simulink model "buck_boost_model"  (R2022a)
settings: Solver=VariableStepAuto  StartTime=0.0  StopTime=0.007  RelTol=1e-3  AbsTol=1e-3
undefined symbols (not defined in the file or in its folder): dutyCycleTs, init_action
libraries: fl_lib x5, nesl_utility x5, ee_lib x3, checkpacklib x1, dspmathops x1, simulink x1, rllib x1
settings Model: Creator=kevin  LastModifiedBy=kevin
settings SolverCC: AutoScaleAbsTol=off  MaxConsecutiveMinStep=2  AlgebraicLoopSolver=TrustRegion
settings DataIOCC: SaveOutput=off  SignalLogging=off  DSMLogging=off  SaveTime=off  ReturnWorkspaceOutputs=off
settings DebuggingCC: UnconnectedInputMsg=warning  UnconnectedOutputMsg=warning  UnconnectedLineMsg=warning  SymbolicDimsDataTypeCodeGenerationDiagnostic=none  SFMachineParentedDataDiag=warning
settings SFSimCC: CustomCodeUndefinedFunction=UseInterfaceOnly
settings RTWCC: DLArmComputeVersion=19.05
settings SimscapeCC: SimscapeLogSimulationStatistics=on  SimscapeLogDataHistory=10000

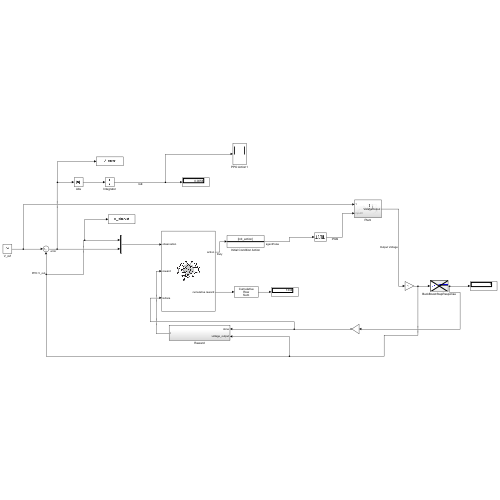
[thumbnail: Simulink's stored preview of the top-level diagram]
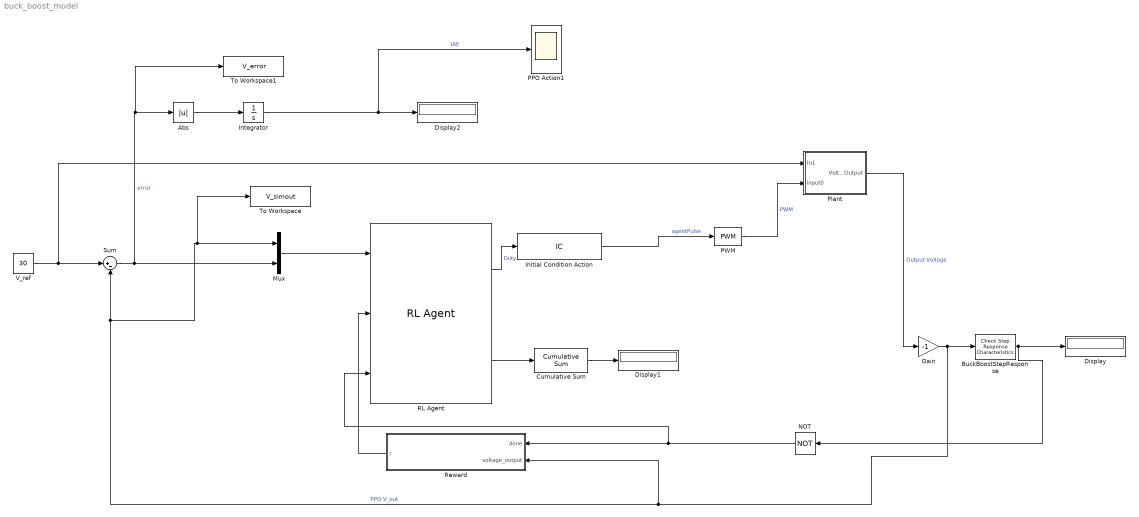
== system buck_boost_model ==
  Abs : Abs  SaturateOnIntegerOverflow=off
  BuckBoostStepResponse : checkpacklib/Check Step Response  Characteristics  InstantiateOnLoad=on  enabled=off  stopWhenAssertionFail=off  export=on  ViewDlgPos=[1.8 41.8 766.4 740.8]  OpenViewOnLoad=off  LaunchViewOnOpen=off  TimeUnits=seconds  EnableStepResponseBound=on  InitialValue=0  FinalValue=30  StepTime=0  RiseTime=0.007  PercentRise=50  SettlingTime=0.0071  PercentSettling=2  PercentOvershoot=30  PercentUndershoot=2
      settings: SourceProductBaseCode=MT,CT,ID,SO
  Cumulative Sum : dspmathops/Cumulative Sum  dim=Rows  InputProcessing=Columns as channels (frame based)  reset_popup=None  roundingMode=Floor  overflowMode=off  outputDataTypeStr=Inherit: Same as accumulator  outputMin=[]  outputMax=[]  outputLastDataTypeStr=Inherit: Same as accumulator
  Display : Display
  Display1 : Display
  Display2 : Display
  Gain : Gain  Gain=-1
  Initial Condition Action : InitialCondition  Value=init_action
  Integrator : Integrator
  Mux : Mux  Inputs=2
  NOT : Logic  Operator=NOT  IconShape=distinctive  AllPortsSameDT=off  OutDataTypeStr=boolean
  PPO Action1 : Scope
  PWM : simulink/Discontinuities/PWM  DisableCoverage=on  Period=1/100000  DisallowZeroDutyCycle=on  RunAtFixedTimeIntervals=off  SampleTime=dutyCycleTs
  Plant : Subsystem
  RL Agent : rllib/RL Agent  Agent=agent  ExternalActionAsInput=off  ProvideLastAction=off  ProvideCumRwd=on  TreatAsDirectFeedthrough=on  UseStrictObservationDataTypes=off
  Reward : Subsystem
  Sum : Sum  Inputs=|+-
  To Workspace : ToWorkspace  VariableName=V_simout  SaveFormat=Timeseries  SampleTime=-1
  To Workspace1 : ToWorkspace  VariableName=V_error  SaveFormat=Timeseries  SampleTime=-1
  V_ref : Constant  Value=30
  wires:
  Plant/1(VoltageOutput) -> Gain/1  "Output Voltage"
  V_ref/1 -> Plant/1(In1), Sum/1
  Mux/1 -> RL Agent/1
  Gain/1 -> To Workspace/1, Mux/1, Sum/2, Reward/2(voltage_output), BuckBoostStepResponse/1  "PPO V_out"
  Sum/1 -> To Workspace1/1, Abs/1, Mux/2  "error"
  Reward/1(r) -> RL Agent/2
  NOT/1 -> Reward/1(done), RL Agent/3
  RL Agent/1 -> Initial Condition Action/1  "Duty"
  RL Agent/2 -> Cumulative Sum/1
  Cumulative Sum/1 -> Display1/1
  Initial Condition Action/1 -> PWM/1  "agentPulse"
  PWM/1 -> Plant/2(input0)  "PWM"
  BuckBoostStepResponse/1 -> NOT/1, Display/1
  Abs/1 -> Integrator/1
  Integrator/1 -> PPO Action1/1, Display2/1  "IAE"

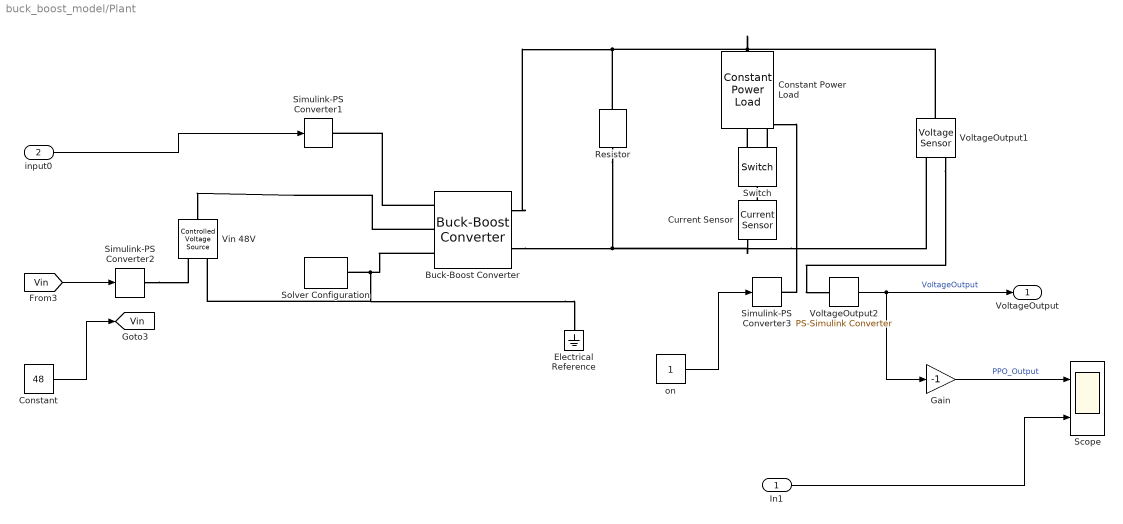
== system buck_boost_model/Plant ==
  In1 : Inport
  input0 : Inport  Port=2
  Buck-Boost Converter : ee_lib/Semiconductors & Converters/Converters/Buck-Boost Converter  device_type=ee.enum.converters.switchingdevice.mosfet  Vf=0.8 V  Ron=0.001 Ohm  Rds=1e-3 Ohm  Goff=1e-3 1/Ohm  Vth=0.0001 V  Vgt=1 V  Vgt_off=-1 V  Ih=1 A  diode_param=ee.enum.converters.diode.nodynamics  diode_Vf=0.00001 V  diode_Ron=1e-3 Ohm  diode_Goff=1e-5 1/Ohm  diode_C=50 nF  diode_iRM=-235 A  diode_iF=300 A  diode_idot=-50 A/us  diode_trr_param=ee.enum.converters.diodetrr.trr_factor  diode_trr_factor=3  diode_trr=15 us  diode_Qrr=1500 s*uA  Lf=34 uH  Rl=0 Ohm  Cf=106 uF  Rf=0.0001 Ohm  snubber_type=ee.enum.converters.snubber.exclude  Rs=0.1 Ohm  Cs=1e-7 F  iL_specify=off  iL_priority=High  iL=0.1 A  iL_nominal_specify=off  iL_nominal_unit=A  iL_nominal_value=1  vc_specify=off  vc_priority=High  vc=0.1 V  vc_nominal_specify=off  vc_nominal_unit=V  vc_nominal_value=1
      settings: SourceProductBaseCode=PS  InternalSimscapePortConfiguration="{\"Bottom\":[],\"Left\":[{\"id\":\"G\",\"label\":\"G\",\"type\":\"input\"},{\"id\":\"p1\",\"label\":\"1+\",\"type\":\"foundation.electrical.electrical\"},{\"id\":\"n1\",\"label\":\"1-\",\"type\":\"foundation.electrical.electrical\"}],\"Right\":[{\"id\":\"p2\",\"label\":\"2+\",\"type\":\"foundation.electrical.electrical\"},{\"id\":\"n2\",\"label\":\"2-\",\"type\":\"foundation.electrical.electrical\"}],\"Top\":[]}"
  Constant : Constant  Value=48
  Constant Power Load : ee_lib/Passive/Constant Power Load  load_type=ee.enum.dc_ac.dc  consumed_power=350 W  min_supply_voltage=25 V  G_reverse=1e-7 S  deltaV=1e-7 V  active_power=500 W  reactive_power=0 V*A  f0=60 Hz  Vrms_min=200 V  enable_fault=simscape.enum.onoff.off  fault_action=simscape.enum.assert.action.none  t_fault=1 s  open_conductance=1e-4 S
      settings: SourceProductBaseCode=PS  InternalSimscapePortConfiguration="{\"Bottom\":[],\"Left\":[{\"id\":\"p\",\"label\":\"+\",\"type\":\"foundation.electrical.electrical\"}],\"Right\":[{\"id\":\"n\",\"label\":\"-\",\"type\":\"foundation.electrical.electrical\"}],\"Top\":[]}"
  Current Sensor : fl_lib/Electrical/Electrical Sensors/Current Sensor
      settings: SourceProductBaseCode=PW,SS,VE
  Electrical Reference : fl_lib/Electrical/Electrical Elements/Electrical Reference
      settings: SourceProductBaseCode=PW,SS,VE
  Gain : Gain  Gain=-1
  Resistor : ee_lib/Passive/Resistor  R=3.6 Ohm  enable_R_tol=0  R_tol=1  tol_distribution=1  nSigma=4  enable_operating_limits=0  operating_limit_action=2  max_working_voltage=100 V  power_rating=1 W  enable_faults=0  fault_action=1  R_faulted=inf Ohm  enable_temporal_fault=0  t_fault=1 s  enable_behavioral_fault=0  max_permissible_current=1 A  t_fail_on_current=1 s  noise_mode=0  sample_time=1e-3 s  repeatability=1  auto_seed=3736368283  user_seed=0  Tdevice=25 degC  power_derating_T1=70 degC  power_derating_T2=155 degC  operating_temperature_range_vec=[-50, 150] degC  alpha=3.93e-3 1/K  Tmeas=25 degC  thermal_mass=100 J/K  temperature_specify=off  temperature_priority=High  temperature=298.15 K  temperature_nominal_specify=off  temperature_nominal_unit=K  temperature_nominal_value=1
  Scope : Scope  NumInputPorts=2
  Simulink-PS Converter1 : nesl_utility/Simulink-PS Converter  PhysicalDomain=network_engine_domain  SubClassName=ps_input  LeftPortType=input  RightPortType=output  PseudoPeriodic=off  Frequencies=[]  NoiseDistribution=none  NoiseParameters=[]  Unit=1  AffineConversion=off  FilteringAndDerivatives=provide  SimscapeFilterOrder=1  InputFilterTimeConstant=0.001  UdotUserProvided=0
      settings: SourceProductBaseCode=SS,PW,VE
  Simulink-PS Converter2 : nesl_utility/Simulink-PS Converter  PhysicalDomain=network_engine_domain  SubClassName=ps_input  LeftPortType=input  RightPortType=output  PseudoPeriodic=off  Frequencies=[]  NoiseDistribution=none  NoiseParameters=[]  Unit=1  AffineConversion=off  FilteringAndDerivatives=zero  SimscapeFilterOrder=1  InputFilterTimeConstant=0.001  UdotUserProvided=0
      settings: SourceProductBaseCode=SS,PW,VE
  Simulink-PS Converter3 : nesl_utility/Simulink-PS Converter  PhysicalDomain=network_engine_domain  SubClassName=ps_input  LeftPortType=input  RightPortType=output  PseudoPeriodic=off  Frequencies=[]  NoiseDistribution=none  NoiseParameters=[]  Unit=1  AffineConversion=off  FilteringAndDerivatives=zero  SimscapeFilterOrder=1  InputFilterTimeConstant=0.001  UdotUserProvided=0
      settings: SourceProductBaseCode=SS,PW,VE
  Solver Configuration : nesl_utility/Solver Configuration  PhysicalDomain=network_engine_domain  SubClassName=solver  LeftPortType=input  RightPortType=generic  Tones=[]  Harmonics=[]  SimulateNoise=off  Profile=off  UseLocalSampling=off  EnableSwitchedLinearOptims=on  FrequencyDomain=off  UseCCode=off  RelTol=0.001  AbsTol=1e-06  MinStep=1e-09  ToWorkspace=off  RevertToSquareIcSolve=off  NumHomotopyIterations=100  PhasorMode=off  PhasorModeNumHarmonics=1  IndexReductionMethod=DerivativeReplacement  DoDC=off  ResidualTolerance=1e-09  UseLocalSolver=off  LocalSolverChoice=NE_BACKWARD_EULER_ADVANCER  LocalSolverSampleTime=0.001  DoFixedCost=off  MaxNonlinIter=3  MaxModeIter=2  ComputeImpulses=off  ImpulseIterations=1  LinearAlgebra=Sparse  LinearAlgebraNumThread=0  EquationFormulation=NE_TIME_EF  DelaysMemoryBudget=1024  AutomaticFiltering=on  FilteringTimeConstant=0.001  PartitionStorageMethod=AS_NEEDED  PartitionMemoryBudget=1024  PartitionMethod=FAST
      settings: SourceProductBaseCode=SS,PW,VE
  Switch : fl_lib/Electrical/Electrical Elements/Switch  R_closed=0.01 Ohm  G_open=1e-8 1/Ohm  Threshold=0.5  i_specify=off  i_priority=None  i=0 A  i_nominal_specify=off  i_nominal_unit=A  i_nominal_value=1  v_specify=off  v_priority=None  v=0 V  v_nominal_specify=off  v_nominal_unit=V  v_nominal_value=1
      settings: SourceProductBaseCode=PW,SS,VE
  Vin 48V : fl_lib/Electrical/Electrical Sources/Controlled Voltage Source
      settings: SourceProductBaseCode=PW,SS,VE
  VoltageOutput1 : fl_lib/Electrical/Electrical Sensors/Voltage Sensor
      settings: SourceProductBaseCode=PW,SS,VE
  VoltageOutput2 : nesl_utility/PS-Simulink Converter  PhysicalDomain=network_engine_domain  SubClassName=ps_output  LeftPortType=input  RightPortType=output  PseudoPeriodic=off  Frequencies=[]  VectorFormat=1-D array  Unit=1  AffineConversion=off
      settings: SourceProductBaseCode=SS,PW,VE
  on : Constant
  VoltageOutput : Outport
  tag scope: Vin=global
  wires:
  [Vin] -> Simulink-PS Converter2/1
  input0/1 -> Simulink-PS Converter1/1
  Constant/1 -> [Vin]
  VoltageOutput2/1 -> Gain/1, VoltageOutput/1  "VoltageOutput"
  on/1 -> Simulink-PS Converter3/1
  In1/1 -> Scope/2
  Gain/1 -> Scope/1  "PPO_Output"
  connections:
  Simulink-PS Converter2/RConn1 -- Vin 48V/RConn1
  Buck-Boost Converter/LConn1 -- Simulink-PS Converter1/RConn1
  Buck-Boost Converter/LConn2 -- Vin 48V/LConn1
  VoltageOutput1/RConn1 -- VoltageOutput2/LConn1
  Buck-Boost Converter/LConn3 -- Electrical Reference/LConn1 -- Solver Configuration/RConn1 -- Vin 48V/RConn2
  Resistor/LConn1 -- Current Sensor/RConn2 -- VoltageOutput1/RConn2 -- Buck-Boost Converter/RConn2
  VoltageOutput1/LConn1 -- Buck-Boost Converter/RConn1 -- Resistor/RConn1 -- Constant Power Load/RConn1
  Switch/RConn2 -- Constant Power Load/LConn1
  Switch/RConn1 -- Simulink-PS Converter3/RConn1
  Current Sensor/LConn1 -- Switch/LConn1

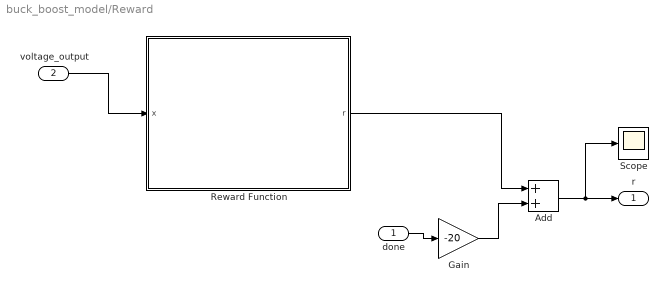
== system buck_boost_model/Reward ==
  done : Inport
  voltage_output : Inport  Port=2
  Add : Sum
  Gain : Gain  Gain=-20
  Reward Function : MATLAB Function  TreatAsAtomicUnit=on
  Scope : Scope
  r : Outport
  wires:
  voltage_output/1 -> Reward Function/1(x)
  Add/1 -> Scope/1, r/1
  done/1 -> Gain/1
  Gain/1 -> Add/2
  Reward Function/1(r) -> Add/1

== matlab function buck_boost_model/Reward/Reward Function ==
  data: x input; r output
function r  = fcn(x)
V_ref = 30;
lower_error_threshold = 0.02;
upper_error_threshold = 0.02;
abs_Vout = abs(x);
error = V_ref - abs_Vout;
abs_error = abs(error);


V_ref_lowerBound = V_ref - (V_ref*lower_error_threshold);
V_ref_upperBound = V_ref + (V_ref*upper_error_threshold);



if ((abs_Vout>V_ref_lowerBound) && ((abs_Vout<V_ref_upperBound)))
    r= 2; 
elseif ((abs_Vout<V_ref_lowerBound))
    r=   (abs_Vout/V_ref)-1;
elseif  ((abs_Vout>V_ref_upperBound))
   r=  1-(abs_Vout/V_ref);
else
    r=0;
end
